simulink library "visionanalysis"  (R2024b)
settings: Solver=ode45  StartTime=0.0  StopTime=10.0  RelTol=1e-3
undefined symbols (not defined in the file or in its folder): dtInfo, fspecial
libraries: visionstatistics x1
(part 1 of 2)
settings Model: Creator=The MathWorks, Inc.  LastModifiedBy=The MathWorks, Inc.
settings SolverCC: AlgebraicLoopSolver=TrustRegion  MaxZcPerStep=1
settings DataIOCC: LimitDataPoints=on  SaveFormat=Array  SignalLoggingSaveFormat=ModelDataLogs  ReturnWorkspaceOutputs=off
settings OptimizationCC: BlockReduction=off  BooleanDataType=off  ReuseModelBlockBuffer=off  ExpressionDepthLimit=2147483647  EfficientMapNaN2IntZero=off  LifeSpan=inf
settings DebuggingCC: SaveWithParameterizedLinksMsg=none  UnderspecifiedInitializationDetection=Classic  MergeDetectMultiDrivingBlocksExec=none  SignalResolutionControl=TryResolveAllWithWarning  FcnCallInpInsideContextMsg=warning  UnconnectedInputMsg=warning  UnconnectedOutputMsg=warning  UnconnectedLineMsg=warning  AllowSymbolicDim=off  StateNameClashWarn=warning  SFUnexpectedBacktrackingDiag=warning  SFNoUnconditionalDefaultTransitionDiag=warning  SFExecutionAtInitializationDiag=none  ArithmeticOperatorsInVariantConditions=warning
settings HardwareCC: ProdBitPerPointer=32  ProdBitPerSizeT=32  ProdBitPerPtrDiffT=32  ProdLargestAtomicFloat=None  ProdIntDivRoundTo=Undefined  ProdEndianess=Unspecified  ProdWordSize=32  ProdHWDeviceType=32-bit Generic  TargetUnknown=on
settings ModelReferenceCC: EnableRefExpFcnMdlSchedulingChecks=on  PropagateSignalLabelsOutOfModel=off
settings SFSimCC: SimUseLocalCustomCode=off
settings RTWCC: RTWUseLocalCustomCode=off  GPUComputeCapability=3.5  DLArmComputeVersion=19.05
settings CodeAppCC: StateflowObjectComments=on
settings GRTTargetCC: TargetLangStandard=C89/C90 (ANSI)  CombineOutputUpdateFcns=off  GRTInterface=on
settings ConfigComp: CovMetricSettings=dw  CovSaveCumulativeToWorkspaceVar=on  CovSaveSingleToWorkspaceVar=on  CovExternalEMLEnable=off  CovSFcnEnable=off

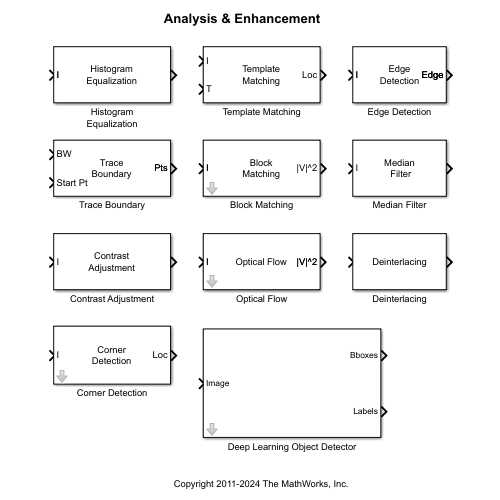
[thumbnail: Simulink's stored preview of the top-level diagram]
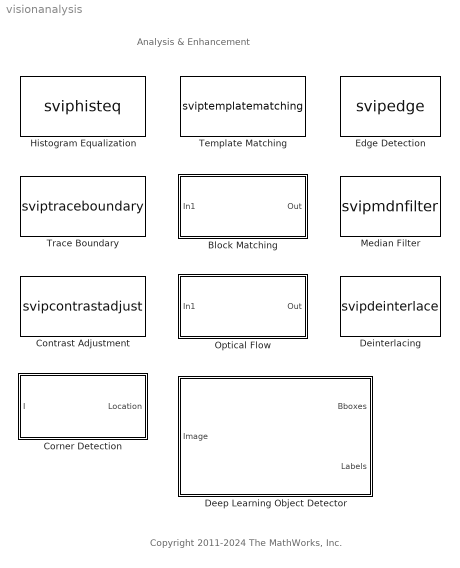
== system visionanalysis ==
  note: Analysis & Enhancement
  note: Copyright 2011-2024 The MathWorks, Inc.
  Block Matching : Subsystem  mask(Block Matching){which2img=Current frame and N-th frame back, N=1, searchMethod=Exhaustive, matchCriteria=Mean square error (MSE), blockSize=[17 17], overlapping=[0 0], maxDisplacement=[7 7], outVelForm=Magnitude-squared, roundingMode=Floor, overflowMode=on, prodOutputMode=Binary point scaling, prodOutputWordLength=32, prodOutputFracLength=0, accumMode=Binary point scaling, accumWordLength=32, accumFracLength=0, outputMode=Binary point scaling, outputWordLength=8, outputFracLength=0, LockScale=off}
      mask prompts: which2img "vision:masks:EstimateMotionBetween"; N "vision:masks:N"; searchMethod "vision:masks:SearchMethod"; matchCriteria "vision:masks:BlockMatchingCriteria"; blockSize "vision:masks:BlockSizeheightWidth"; overlapping "vision:masks:OverlapSizerC"; maxDisplacement "vision:masks:MaximumDisplacementrC"; outVelForm "vision:masks:VelocityOutput"; roundingMode "vision:masks:RoundingMode"; overflowMode "vision:masks:SaturateOnIntegerOverflow"; LockScale "Simulink:masks:LockDataTypeAgainstFxpTools_MP"
      mask help: vision:masks:BlockMatchingDescription
      mask init:
      | [disp_str,si,so]=vipblkblockmatch('icon',which2img);
      | vipblkblockmatch('init');
      mask Help: eval('visionblockhelp');
      mask TypeOptions which2img: vision:masks:TwoImages | vision:masks:CurrentFrameAndNthFrameBack
      mask Callback which2img: vipblkblockmatch('dynamic');
      mask TypeOptions searchMethod: vision:masks:Exhaustive | vision:masks:Threestep
      mask TypeOptions matchCriteria: vision:masks:MeanSquareErrorMSE | vision:masks:MeanAbsoluteDifferenceMAD
      mask Callback matchCriteria: vipblkblockmatch('dynamic');
      mask TypeOptions outVelForm: vision:masks:HorizontalAndVerticalComponentsI | vision:masks:Magnitudesquared
      mask Callback outVelForm: vipblkblockmatch('dynamic');
      mask TypeOptions roundingMode: Simulink:dialog:Ceiling_CB | Simulink:dialog:Convergent_CB | Simulink:dialog:Floor_CB | Simulink:dialog:Nearest_CB | Simulink:dialog:Round_CB | Simulink:dialog:Simplest_CB | Simulink:dialog:Zero_CB
      mask TypeOptions prodOutputMode: Simulink:dialog:UDTSameAsInputRule | vision:masks:BinaryPointScaling
      mask Callback prodOutputMode: vipblkblockmatch('dynamic');
      mask TypeOptions accumMode: vision:masks:BinaryPointScaling
      mask Callback accumMode: vipblkblockmatch('dynamic');
      mask TypeOptions outputMode: vision:masks:BinaryPointScaling
      mask Callback outputMode: vipblkblockmatch('dynamic');
      mask DialogControl MainTab Prompt: vision:masks:Main
      mask DialogControl which2img Prompt: Estimate motion between:
      mask DialogControl N Prompt: N:
      mask DialogControl searchMethod Prompt: Search method:
      mask DialogControl matchCriteria Prompt: Block matching criteria:
      mask DialogControl blockSize Prompt: Block size [height width]:
      mask DialogControl overlapping Prompt: Overlap size [r c]:
      mask DialogControl maxDisplacement Prompt: Maximum displacement [r c]:
      mask DialogControl outVelForm Prompt: Velocity output:
      mask DialogControl DataTypesTab Prompt: Simulink:dialog:DataTypesTab
      mask DialogControl FloatingPointTrumpRule Prompt: Simulink:dialog:FloatingPointTrumpRule
      mask DialogControl FixPtOpParamsGroupBox Prompt: vision:masks:FixptOpParams
      mask DialogControl roundingMode Prompt: Rounding mode:
      mask DialogControl overflowMode Prompt: Saturate on integer overflow
      mask DialogControl FixptDatatypesGroupBox Prompt: vision:masks:FixptDataTypes
      mask DialogControl DataTypeColumnLabel Prompt: Simulink:dialog:FcnColumnHeaderDataType
      mask DialogControl SignedColumnLabel Prompt: Simulink:dialog:UDTSignedSign
      mask DialogControl WordLengthColumnLabel Prompt: Simulink:dialog:UDTWordLengthEdit
      mask DialogControl FractionLengthColumnLabel Prompt: Simulink:dialog:UDTFractionLengthEdit
      mask DialogControl prodOutputLabel Prompt: Simulink:dialog:ProdPrompt
      mask DialogControl prodOutputSignedText Prompt: Simulink:dialog:yes_CB
      mask DialogControl accumLabel Prompt: Simulink:dialog:AccumPrompt
      mask DialogControl accumSignedText Prompt: dspshared:FixptDialog:yes
      mask DialogControl outputLabel Prompt: Simulink:dialog:OutputPrompt
      mask DialogControl outputSignedText Prompt: Simulink:dialog:no_CB
      mask DialogControl LockScale Prompt: Lock data type settings against changes by the fixed-point tools
      mask Display:
      | disp(disp_str);
      | port_label('input',si(1).port,si(1).txt);
      | port_label('input',si(2).port,si(2).txt);
      | 
      | port_label('output',1,so(1).txt);
  Contrast Adjustment : S-Function  FunctionName=svipcontrastadjust  Parameters=methodInputRange, rangeIn, fracSaturate, isBinNum, binNum, methodOutputRange, rangeOut, prod1Mode, prod1WordLength, prod1FracLength, prod2Mode, prod2WordLength, prod2FracLength, dtInfo.roundingMode, dtInfo.overflowMode  SFunctionDeploymentMode=off  EnableBusSupport=off  mask(Contrast Adjustment){methodInputRange=Full input data range [min max], rangeIn=[0 255], fracSaturate=[1 1], isBinNum=on, binNum=256, methodOutputRange=Full data type range, rangeOut=[0 255], roundingMode=Floor, overflowMode=off, prod1Mode=Binary point scaling, prod1WordLength=32, prod1FracLength=16, prod2Mode=Binary point scaling, prod2WordLength=32, prod2FracLength=16, LockScale=off}
      mask prompts: methodInputRange "vision:masks:AdjustPixelValuesFrom"; rangeIn "vision:masks:RangelowHigh"; fracSaturate "vision:masks:PercentageOfPixelsToSaturatelowH"; isBinNum "vision:masks:SpecifyNumberOfHistogramBinsused"; binNum "vision:masks:NumberOfHistogramBins"; methodOutputRange "vision:masks:AdjustPixelValuesTo"; rangeOut "vision:masks:RangelowHigh"; roundingMode "vision:masks:RoundingMode"; overflowMode "vision:masks:SaturateOnIntegerOverflow"; LockScale "Simulink:masks:LockDataTypeAgainstFxpTools_MP"
      mask help: vision:masks:ContrastAdjustmentDescription
      mask init:
      | dtInfo = dspGetFixptDataTypeInfo(gcbh,1);
      | fracSaturate = single(fracSaturate) ./ single(100);
      mask Help: eval('visionblockhelp');
      mask TypeOptions methodInputRange: vision:masks:FullInputDataRangeminMax | vision:masks:UserdefinedRange | vision:masks:RangeDeterminedBySaturating
      mask Callback methodInputRange: vipblkcontrast;
      mask Callback isBinNum: vipblkcontrast;
      mask TypeOptions methodOutputRange: vision:masks:FullDataTypeRange | vision:masks:UserdefinedRange
      mask Callback methodOutputRange: vipblkcontrast;
      mask TypeOptions roundingMode: Simulink:dialog:Ceiling_CB | Simulink:dialog:Convergent_CB | Simulink:dialog:Floor_CB | Simulink:dialog:Nearest_CB | Simulink:dialog:Round_CB | Simulink:dialog:Simplest_CB | Simulink:dialog:Zero_CB
      mask TypeOptions prod1Mode: vision:masks:BinaryPointScaling
      mask Callback prod1Mode: vipblkcontrast;
      mask TypeOptions prod2Mode: vision:masks:BinaryPointScaling
      mask Callback prod2Mode: vipblkcontrast;
      mask DialogControl mainTab Prompt: vision:masks:Main
      mask DialogControl methodInputRange Prompt: Adjust pixel values from:
      mask DialogControl rangeIn Prompt: Range [low high]:
      mask DialogControl fracSaturate Prompt: Percentage of pixels to saturate [low high]:
      mask DialogControl isBinNum Prompt: Specify number of histogram bins (used to calculate the range when outliers are eliminated)
      mask DialogControl binNum Prompt: Number of histogram bins:
      mask DialogControl methodOutputRange Prompt: Adjust pixel values to:
      mask DialogControl rangeOut Prompt: Range [low high]:
      mask DialogControl dataTypesTab Prompt: vision:masks:DataTypes
      mask DialogControl dataTypesDescription Prompt: Simulink:dialog:FloatingPointTrumpRule
      mask DialogControl fixedptOpParams Prompt: vision:masks:FixptOpParams
      mask DialogControl roundingMode Prompt: Rounding mode:
      mask DialogControl overflowMode Prompt: Saturate on integer overflow
      mask DialogControl fixedptDataTypes Prompt: vision:masks:FixptDataTypes
      mask DialogControl openDataTypeDiagram Prompt: vision:masks:OpenDataTypeDiagram
      mask DialogControl openDataTypeDiagram Callback: uiservices.helpview('$DOCROOT$\toolbox\vision\vision.map', 'contrastadjust', 'CSHelpWindow')
      mask DialogControl dataTypeColoumnLabel Prompt: Simulink:dialog:FcnColumnHeaderDataType
      mask DialogControl signedColoumnLabel Prompt: Simulink:dialog:UDTSignedSign
      mask DialogControl wordLegthColoumnlabel Prompt: Simulink:dialog:UDTWordLengthEdit
      mask DialogControl fracLengthColumnLabel Prompt: Simulink:dialog:UDTFractionLengthEdit
      mask DialogControl product1Label Prompt: vision:masks:Product1
      mask DialogControl prod1SignedText Prompt: Simulink:dialog:yes_CB
      mask DialogControl product2Label Prompt: vision:masks:Product2
      mask DialogControl prod2SignedText Prompt: Simulink:dialog:yes_CB
      mask DialogControl LockScale Prompt: Lock data type settings against changes by the fixed-point tools
      mask Display:
      | disp('Contrast\nAdjustment');
      | port_label('input',1,'I');
  Corner Detection : Subsystem  mask(Corner Detection){method=Harris corner detection (Harris & Stephens), factor=0.04, filter=fspecial('gaussian', [1 5], 1.5), thrInten=0.1, thrAngle=157.5, output=Obsolete9b, outputInUse=Corner location, maxNum=200, thrMetric=0.0005, neighborSize=[11 11], isOutVarDim=on, roundingMode=Floor, overflowMode=off, firstCoeffMode=Specify word length, firstCoeffWordLength=16, firstCoeffFracLength=16, prodOutputMode=Binary point scaling, prodOutputWordLength=32, prodOutputFracLength=0, accumMode=Binary point scaling, accumWordLength=32, accumFracLength=0, memoryMode=Binary point scaling, memoryWordLength=32, memoryFracLength=0, outputMode=Same as accumulator, outputWordLength=32, outputFracLength=0, LockScale=off}
      mask prompts: method "vision:masks:Method"; factor "vision:masks:SensitivityFactor"; filter "vision:masks:CoefficientsSeparableSmoothing"; thrInten "vision:masks:IntensityComparisonThreshold"; thrAngle "vision:masks:MaximumAngleToBeConsidered"; output "dspshared:FixptDialog:Output_MP"; outputInUse "dspshared:FixptDialog:Output_MP"; maxNum "vision:masks:MaximumNumberOfCorners"; thrMetric "vision:masks:MinimumMetricValueThatIndicates"; neighborSize "vision:masks:NeighborhoodSizesuppressRegion"; isOutVarDim "vision:masks:OutputVariableSizeSignal"; roundingMode "vision:masks:RoundingMode"; overflowMode "vision:masks:SaturateOnIntegerOverflow"; LockScale "Simulink:masks:LockDataTypeAgainstFxpTools_MP"
      mask help: vision:masks:CornerDetectionDescription
      mask init:
      | blkh = gcbh;
      | dtInfo = dspGetFixptDataTypeInfo(blkh, 63); %63
      | outport = vipblkcornerdetection(blkh, output, outputInUse, isOutVarDim);
      mask Help: eval('visionblockhelp');
      mask TypeOptions method: vision:masks:HarrisCornerDetectionHarrisSteph | vision:masks:MinimumEigenvalueShiTomasi | vision:masks:LocalIntensityComparisonRosenDr
      mask Callback method: vipblkcddynamic;
      mask TypeOptions thrAngle: 22.5 | 45.0 | 67.5 | 90.0 | 112.5 | 135.0 | 157.5
      mask TypeOptions output: vision:masks:CornerLocation | vision:masks:CornerLocationAndMetricMatrix | vision:masks:MetricMatrix | vision:masks:Obsolete9b
      mask TypeOptions outputInUse: vision:masks:CornerLocation | vision:masks:CornerLocationAndMetricMatrix | vision:masks:MetricMatrix
      mask Callback outputInUse: vipblkcddynamic;
      mask TypeOptions roundingMode: Simulink:dialog:Ceiling_CB | Simulink:dialog:Convergent_CB | Simulink:dialog:Floor_CB | Simulink:dialog:Nearest_CB | Simulink:dialog:Round_CB | Simulink:dialog:Simplest_CB | Simulink:dialog:Zero_CB
      mask TypeOptions firstCoeffMode: Simulink:dialog:UDTSameAsInputWordLengthRule | vision:masks:SpecifyWordLength | vision:masks:BinaryPointScaling
      mask Callback firstCoeffMode: vipblkcddynamic;
      mask TypeOptions prodOutputMode: Simulink:dialog:UDTSameAsInputRule | vision:masks:BinaryPointScaling
      mask Callback prodOutputMode: vipblkcddynamic;
      mask TypeOptions accumMode: Simulink:dialog:UDTSameAsInputRule | vision:masks:BinaryPointScaling
      mask Callback accumMode: vipblkcddynamic;
      mask TypeOptions memoryMode: Simulink:dialog:UDTSameAsInputRule | vision:masks:BinaryPointScaling
      mask Callback memoryMode: vipblkcddynamic;
      mask TypeOptions outputMode: Simulink:dialog:UDTSameAsAccumulatorRule | Simulink:dialog:UDTSameAsInputRule | vision:masks:BinaryPointScaling
      mask Callback outputMode: vipblkcddynamic;
      mask DialogControl maintab Prompt: vision:masks:Main
      mask DialogControl method Prompt: Method:
      mask DialogControl factor Prompt: Sensitivity factor (0<k<0.25):
      mask DialogControl filter Prompt: Coefficients for separable smoothing filter:
      mask DialogControl thrInten Prompt: Intensity comparison threshold:
      mask DialogControl thrAngle Prompt: Maximum angle to be considered a corner (in degrees):
      mask DialogControl output Prompt: Output:
      mask DialogControl outputInUse Prompt: Output:
      mask DialogControl maxNum Prompt: Maximum number of corners:
      mask DialogControl thrMetric Prompt: Minimum metric value that indicates a corner:
      mask DialogControl neighborSize Prompt: Neighborhood size (suppress region around detected corners):
      mask DialogControl isOutVarDim Prompt: Output variable size signal
      mask DialogControl dataTypesTab Prompt: vision:masks:DataTypes
      mask DialogControl fixptTrumpRule Prompt: Simulink:dialog:FloatingPointTrumpRule
      mask DialogControl fixptOpParams Prompt: vision:masks:FixptOpParams
      mask DialogControl roundingMode Prompt: Rounding mode:
      mask DialogControl overflowMode Prompt: Saturate on integer overflow
      mask DialogControl fixptDataTypes Prompt: vision:masks:FixptDataTypes
      mask DialogControl openDataTypeDiagram Prompt: vision:masks:OpenDataTypeDiagram
      mask DialogControl openDataTypeDiagram Callback: uiservices.helpview('$DOCROOT$\toolbox\vision\vision.map', 'cornerdetection', 'CSHelpWindow')
      mask DialogControl dataTypeColumnLabel Prompt: Simulink:dialog:FcnColumnHeaderDataType
      mask DialogControl signedColumnLabel Prompt: Simulink:dialog:UDTSignedSign
      mask DialogControl wordLengthColumnLabel Prompt: Simulink:dialog:UDTWordLengthEdit
      mask DialogControl fractionLengthColumnLabel Prompt: Simulink:dialog:UDTFractionLengthEdit
      mask DialogControl firstCoeffLabel Prompt: vision:masks:Coefficients
      mask DialogControl firstCoeffSignedText Prompt: Simulink:dialog:Yes_CB
      mask DialogControl prodOutputLabel Prompt: vision:masks:ProductOutput
      mask DialogControl prodOutputSignedText Prompt: Simulink:dialog:Yes_CB
      mask DialogControl accumLabel Prompt: vision:masks:Accumulator
      mask DialogControl accumSignedText Prompt: Simulink:dialog:Yes_CB
      mask DialogControl memoryLabel Prompt: vision:masks:Memory
      mask DialogControl memorySignedText Prompt: Simulink:dialog:Yes_CB
      mask DialogControl outputLabel Prompt: vision:masks:MetricOutput
      mask DialogControl outputSignedText Prompt: Simulink:dialog:Yes_CB
      mask DialogControl LockScale Prompt: Lock data type settings against changes by the fixed-point tools
      mask Display:
      | disp('Corner\nDetection');
      | port_label('input',1,'I');
      | port_label('output', outport(1).port, outport(1).txt);
      | port_label('output', outport(2).port, outport(2).txt);
      | port_label('output', outport(3).port, outport(3).txt);
  Deep Learning Object Detector : Subsystem  mask(Deep Learning Object Detector){Detector=Detector from MAT-file, DetectorFunction=untitled, DetectorFilePath=untitled.mat, MaxDetections=500, Bboxes=on, Labels=on, Scores=off, UseROI=off, AutoResize=on, ROI=[1 1 100 100], Threshold=0.5, NumStrongestRegions=2000, UseMinSize=off, MinSize=[1 1], UseMaxSize=off, MaxSize=[50 50], ForceInterpretedSim=off}
      mask prompts: Detector "vision:ObjectDetectorBlock:Detector"; DetectorFunction "vision:ObjectDetectorBlock:MatlabFunction"; DetectorFilePath "vision:ObjectDetectorBlock:FilePath"; MaxDetections "vision:ObjectDetectorBlock:MaxDetections"; Bboxes "vision:ObjectDetectorBlock:Bboxes"; Labels "vision:ObjectDetectorBlock:Labels"; Scores "vision:ObjectDetectorBlock:Scores"; UseROI "vision:ObjectDetectorBlock:UseROI"; AutoResize "Automatically resize input"; Threshold "vision:ObjectDetectorBlock:Threshold"; NumStrongestRegions "vision:ObjectDetectorBlock:NumStrongestRegions"; UseMinSize "vision:ObjectDetectorBlock:UseMinSize"; UseMaxSize "vision:ObjectDetectorBlock:UseMaxSize"; ForceInterpretedSim "vision:ObjectDetectorBlock:ForceInterpretedSim"
      mask help: vision:ObjectDetectorBlock:Description
      mask init:
      | vision.internal.blocks.objectDetectorBlockWrapper(...
      |     'deep.blocks.internal.configureObjectDetector', ...
      |     gcb, ...
      |     bdroot, ...
      |     Detector, ...
      |     DetectorFilePath, ...
      |     DetectorFunction, ...
      |     logical(UseROI), ...
      |     ROI, ...
      |     Threshold, ...
      |     NumStrongestRegions, ...
      |     logical(AutoResize), ...
      |     logical(UseMinSize), ...
      |     MinSize, ...
      |     logical(UseMaxSize), ...
      |     MaxSize, ...
      |     MaxDetections, ...
      |     logical(Bboxes), ...
      |     logical(Labels), ...
      |     logical(Scores), ...
      |     logical(ForceInterpretedSim));
      mask Help: helpview('vision', 'nnet_model_detect')
      mask TypeOptions Detector: vision:ObjectDetectorBlock:DetectorFromMatFile | vision:ObjectDetectorBlock:DetectorFromFunction
      mask Callback Detector: vision.internal.blocks.objectDetectorBlockWrapper('deep.blocks.internal.setNetworkSelectVisibility',gcb);
      mask Callback DetectorFunction: vision.internal.blocks.objectDetectorBlockWrapper('deep.blocks.internal.setObjectDetectorOptionsVisibility', gcb);
      mask Callback DetectorFilePath: vision.internal.blocks.objectDetectorBlockWrapper('deep.blocks.internal.setObjectDetectorOptionsVisibility', gcb);
      mask Callback UseROI: vision.internal.blocks.objectDetectorBlockWrapper('deep.blocks.internal.setEnabledParameterVisibility', gcb, 'UseROI', 'ROI');
      mask Callback UseMinSize: vision.internal.blocks.objectDetectorBlockWrapper('deep.blocks.internal.setEnabledParameterVisibility', gcb, 'UseMinSize', 'MinSize');
      mask Callback UseMaxSize: vision.internal.blocks.objectDetectorBlockWrapper('deep.blocks.internal.setEnabledParameterVisibility', gcb, 'UseMaxSize', 'MaxSize');
      mask DialogControl Detector Prompt: Detector:
      mask DialogControl DetectorFunction Prompt: MATLAB function:
      mask DialogControl DetectorFilePath Prompt: File path:
      mask DialogControl BrowseButton Prompt: vision:ObjectDetectorBlock:Browse
      mask DialogControl BrowseButton Callback: vision.internal.blocks.objectDetectorBlockWrapper('deep.blocks.internal.handleBrowseButtonClick', gcb);
      mask DialogControl OutputsTab Prompt: vision:ObjectDetectorBlock:Outputs
      mask DialogControl OutputsSizeGroup Prompt: vision:ObjectDetectorBlock:OutputsSize
      mask DialogControl MaxDetections Prompt: Maximum number of detections:
      mask DialogControl OutputPortsGroup Prompt: vision:ObjectDetectorBlock:OutputPorts
      mask DialogControl Bboxes Prompt: Bounding boxes
      mask DialogControl AdvancedTab Prompt: vision:ObjectDetectorBlock:Advanced
      mask DialogControl AdvancedParametersGroup Prompt: vision:ObjectDetectorBlock:AdvancedParameters
      mask DialogControl UseROI Prompt: Specify region of interest
      mask DialogControl Threshold Prompt: Detection threshold:
      mask DialogControl NumStrongestRegions Prompt: Number of strongest regions:
      mask DialogControl UseMinSize Prompt: Specify minimum region size
      mask DialogControl UseMaxSize Prompt: Specify maximum region size
      mask DialogControl HiddenContainer Prompt: Hidden Parameters
      mask DialogControl ForceInterpretedSim Prompt: Force interpreted simulation
  Deinterlacing : S-Function  FunctionName=svipdeinterlace  Parameters=method,isInputTransposed,dtInfo.accumMode,dtInfo.accumWordLength,dtInfo.accumFracLength,dtInfo.outputMode,dtInfo.outputWordLength,dtInfo.outputFracLength,dtInfo.roundingMode,dtInfo.overflowMode  SFunctionDeploymentMode=off  EnableBusSupport=off  mask(Deinterlacing){method=Line repetition, isInputTransposed=off, roundingMode=Floor, overflowMode=on, prodOutputMode=Same as input, prodOutputWordLength=12, prodOutputFracLength=3, accumMode=Binary point scaling, accumWordLength=12, accumFracLength=3, outputMode=Same as input, outputWordLength=8, outputFracLength=0, LockScale=off}
      mask prompts: method "vision:masks:Method"; isInputTransposed "vision:masks:InputImageIsTransposed"; roundingMode "vision:masks:RoundingMode"; overflowMode "vision:masks:SaturateOnIntegerOverflow"; LockScale "Simulink:masks:LockDataTypeAgainstFxpTools_MP"
      mask help: vision:masks:DeinterlacingDescription
      mask init:
      | dtInfo = dspGetFixptDataTypeInfo(gcbh,7);
      | vipblkdeinterlacing('dynamic');
      mask Help: eval('visionblockhelp');
      mask TypeOptions method: vision:masks:LineRepetition | vision:masks:LinearInterpolation | vision:masks:VerticalTemporalMedianFiltering
      mask Callback method: vipblkdeinterlacing('dynamic');
      mask TypeOptions roundingMode: Simulink:dialog:Ceiling_CB | Simulink:dialog:Convergent_CB | Simulink:dialog:Floor_CB | Simulink:dialog:Nearest_CB | Simulink:dialog:Round_CB | Simulink:dialog:Simplest_CB | Simulink:dialog:Zero_CB
      mask TypeOptions prodOutputMode: Simulink:dialog:UDTSameAsInputRule | vision:masks:BinaryPointScaling
      mask Callback prodOutputMode: vipblkdeinterlacing('dynamic');
      mask TypeOptions accumMode: Simulink:dialog:UDTSameAsInputRule | vision:masks:BinaryPointScaling
      mask Callback accumMode: vipblkdeinterlacing('dynamic');
      mask TypeOptions outputMode: Simulink:dialog:UDTSameAsInputRule | vision:masks:BinaryPointScaling
      mask Callback outputMode: vipblkdeinterlacing('dynamic');
      mask DialogControl MainTab Prompt: vision:masks:Main
      mask DialogControl method Prompt: Method:
      mask DialogControl isInputTransposed Prompt: Input image is transposed (data order is row major)
      mask DialogControl DataTypesTab Prompt: Simulink:dialog:DataTypesTab
      mask DialogControl emptyFixpt Prompt: vision:masks:FixedpointParametersLinearInterp
      mask DialogControl FloatingPointTrumpRule Prompt: Simulink:dialog:FloatingPointTrumpRule
      mask DialogControl FixPtOpParamsGroupBox Prompt: dspshared:FixptDialog:fixptOpParams
      mask DialogControl roundingMode Prompt: Rounding mode:
      mask DialogControl overflowMode Prompt: Saturate on integer overflow
      mask DialogControl FixptDatatypesGroupBox Prompt: dspshared:FixptDialog:fixptDataTypes
      mask DialogControl DataTypeColumnLabel Prompt: Simulink:dialog:BreakPointTableHeaderDT
      mask DialogControl SignedColumnLabel Prompt: dspshared:FixptDialog:signed
      mask DialogControl WordLengthColumnLabel Prompt: dspshared:FixptDialog:wordLength
      mask DialogControl FractionLengthColumnLabel Prompt: dspshared:FixptDialog:fractionLength
      mask DialogControl prodOutputLabel Prompt: Simulink:dialog:ProdPrompt
      mask DialogControl prodOutputSignedText Prompt: Simulink:dialog:UDTSameAsInputRule
      mask DialogControl accumLabel Prompt: Simulink:dialog:AccumPrompt
      mask DialogControl accumSignedText Prompt: Simulink:dialog:UDTSameAsInputRule
      mask DialogControl outputLabel Prompt: Simulink:dialog:OutputPrompt
      mask DialogControl outputSignedText Prompt: Simulink:dialog:UDTSameAsInputRule
      mask DialogControl LockScale Prompt: Lock data type settings against changes by the fixed-point tools
      mask Display: disp('Deinterlacing')
  Edge Detection : S-Function  FunctionName=svipedge  Parameters=method, outputType, userDefinedThreshold, thresholdSource, threshold, thresholdTuning, edgeThinning,threshold_canny,autoPercent,sigma,dtInfo. prodOutputMode,dtInfo.prodOutputWordLength,dtInfo.prodOutputFracLength,dtInfo.accumMode,dtInfo.accumWordLength,dtInfo.accumFracLength,dtInfo.outputMode,dtInfo.outputWordLength,dtInfo.outputFracLength,dtInfo.roundingMode,dtInfo.overflowMode  SFunctionDeploymentMode=off  EnableBusSupport=off  mask(Edge Detection){method=Sobel, outputType=Binary image, userDefinedThreshold=off, thresholdSource=Input port, threshold=20, thresholdTuning=4, edgeThinning=off, threshold_canny=[0.25 0.60], autoPercent=70, sigma=1, roundingMode=Floor, overflowMode=off, prodOutputMode=Binary point scaling, prodOutputWordLength=32, prodOutputFracLength=8, accumMode=Same as first input, accumWordLength=32, accumFracLength=8, outputMode=Same as first input, outputWordLength=16, outputFracLength=4, LockScale=off}
      mask prompts: method "vision:masks:Method"; outputType "vision:masks:OutputType"; userDefinedThreshold "vision:masks:UserdefinedThreshold"; thresholdSource "vision:masks:ThresholdSource"; threshold "vision:masks:Threshold"; thresholdTuning "vision:masks:ThresholdScaleFactor"; edgeThinning "vision:masks:EdgeThinning"; threshold_canny "vision:masks:ThresholdLowHigh"; autoPercent "vision:masks:ApproximatePercentageOfWeakEdge"; sigma "vision:masks:StandardDeviationOfGaussian"; roundingMode "vision:masks:RoundingMode"; overflowMode "vision:masks:SaturateOnIntegerOverflow"; LockScale "Simulink:masks:LockDataTypeAgainstFxpTools_MP"
      mask help: vision:masks:EdgeDetectionDescription
      mask init:
      | [si,so,blkname,dtInfo]= vipblkedge('init');
      mask Help: eval('visionblockhelp');
      mask TypeOptions method: vision:masks:Sobel | vision:masks:Prewitt | vision:masks:Roberts | vision:masks:Canny
      mask Callback method: vipblkedge('dynamic');
      mask TypeOptions outputType: vision:masks:BinaryImage | vision:masks:GradientComponents | vision:masks:BinaryImageAndGradientComponents
      mask Callback outputType: vipblkedge('dynamic');
      mask Callback userDefinedThreshold: vipblkedge('dynamic');
      mask TypeOptions thresholdSource: vision:masks:SpecifyViaDialog | vision:masks:InputPort
      mask Callback thresholdSource: vipblkedge('dynamic');
      mask TypeOptions roundingMode: Simulink:dialog:Ceiling_CB | Simulink:dialog:Convergent_CB | Simulink:dialog:Floor_CB | Simulink:dialog:Nearest_CB | Simulink:dialog:Round_CB | Simulink:dialog:Simplest_CB | Simulink:dialog:Zero_CB
      mask TypeOptions prodOutputMode: Simulink:dialog:UDTSameAsFirstInputRule | vision:masks:BinaryPointScaling
      mask Callback prodOutputMode: vipblkedge('dynamic');
      mask TypeOptions accumMode: Simulink:dialog:UDTSameAsProductRule | Simulink:dialog:UDTSameAsFirstInputRule | vision:masks:BinaryPointScaling
      mask Callback accumMode: vipblkedge('dynamic');
      mask TypeOptions outputMode: Simulink:dialog:UDTSameAsAccumulatorRule | Simulink:dialog:UDTSameAsProductRule | Simulink:dialog:UDTSameAsFirstInputRule | vision:masks:BinaryPointScaling
      mask Callback outputMode: vipblkedge('dynamic');
      mask DialogControl MainTab Prompt: vision:masks:Main
      mask DialogControl method Prompt: Method:
      mask DialogControl outputType Prompt: Output type:
      mask DialogControl userDefinedThreshold Prompt: User-defined threshold
      mask DialogControl thresholdSource Prompt: Threshold source:
      mask DialogControl threshold Prompt: Threshold:
      mask DialogControl thresholdTuning Prompt: Threshold scale factor:(used to automatically calculate threshold value)
      mask DialogControl edgeThinning Prompt: Edge thinning
      mask DialogControl threshold_canny Prompt: Threshold, [Low High]:
      mask DialogControl autoPercent Prompt: Approximate percentage of weak edge and nonedge pixels:(used to automatically calculate threshold values)
      mask DialogControl sigma Prompt: Standard deviation of Gaussian filter:
      mask DialogControl DataTypesTab Prompt: Simulink:dialog:DataTypesTab
      mask DialogControl emptyFixpt Prompt: vision:masks:FixedpointInputIsNotSupported
      mask DialogControl FloatingPointTrumpRule Prompt: Simulink:dialog:FloatingPointTrumpRule
      mask DialogControl FixPtOpParamsGroupBox Prompt: dspshared:FixptDialog:fixptOpParams
      mask DialogControl roundingMode Prompt: Rounding mode:
      mask DialogControl overflowMode Prompt: Saturate on integer overflow
      mask DialogControl FixptDatatypesGroupBox Prompt: dspshared:FixptDialog:fixptDataTypes
      mask DialogControl DataTypeColumnLabel Prompt: Simulink:dialog:BreakPointTableHeaderDT
      mask DialogControl SignedColumnLabel Prompt: dspshared:FixptDialog:signed
      mask DialogControl WordLengthColumnLabel Prompt: dspshared:FixptDialog:wordLength
      mask DialogControl FractionLengthColumnLabel Prompt: dspshared:FixptDialog:fractionLength
      mask DialogControl prodOutputLabel Prompt: Simulink:dialog:ProdPrompt
      mask DialogControl prodOutputSignedText Prompt: dspshared:FixptDialog:yes
      mask DialogControl accumLabel Prompt: Simulink:dialog:AccumPrompt
      mask DialogControl accumSignedText Prompt: dspshared:FixptDialog:yes
      mask DialogControl outputLabel Prompt: vision:masks:Gradients
      mask DialogControl outputSignedText Prompt: dspshared:FixptDialog:yes
      mask DialogControl LockScale Prompt: Lock data type settings against changes by the fixed-point tools
      mask Display:
      | disp(blkname)
      | 
      | port_label('input', si(1).port, si(1).txt);
      | port_label('input', si(2).port, si(2).txt);
      | 
      | port_label('output',so(1).port, so(1).txt);
      | port_label('output',so(2).port, so(2).txt);
      | port_label('output',so(3).port, so(3).txt);
  Histogram Equalization : S-Function  FunctionName=sviphisteq  Parameters=specify, numbins, src, hist  SFunctionDeploymentMode=off  EnableBusSupport=off  mask(Histogram Equalization){specify=Uniform, numbins=64, src=Specify via dialog, hist=ones(1,64)}
      mask prompts: specify "vision:masks:TargetHistogram"; numbins "vision:masks:NumberOfBins"; src "vision:masks:HistogramSource"; hist "vision:masks:Histogram"
      mask help: vision:masks:HistogramEqualizationDescription
      mask init:
      | ports(1).num = 1;
      | ports(1).txt = 'I';
      | if (specify == 2 && src == 2)
      | 	ports(2).num = 2;
      | 	ports(2).txt = 'Hist';
      | else
      | 	ports(2).num = 1;
      | 	ports(2).txt = 'I';
      | end
      mask Help: eval('visionblockhelp');
      mask TypeOptions specify: vision:masks:Uniform | vision:masks:Userdefined
      mask Callback specify:
      | if (strcmp(get_param(gcbh,'specify'),'Uniform'))
      | 	set_param(gcbh,'MaskVisibilities',{'on','on','off','off'});
      | else
      | 	if (strcmp(get_param(gcbh,'src'),'Input port'))
      | 		set_param(gcbh,'MaskVisibilities',{'on','off','on','off'});
      | 	else
      | 		set_param(gcbh,'MaskVisibilities',{'on','off','on','on'});
      | 	end
      | end
      mask TypeOptions src: vision:masks:SpecifyViaDialog | vision:masks:InputPort
      mask Callback src:
      | if (strcmp(get_param(gcbh,'specify'),'User-defined'))
      | 	if (strcmp(get_param(gcbh,'src'),'Input port'))
      | 		set_param(gcbh,'MaskVisibilities',{'on','off','on','off'});
      | 	else
      | 		set_param(gcbh,'MaskVisibilities',{'on','off','on','on'});
      | 	end
      | end
      mask Display:
      | disp('Histogram\nEqualization');
      | 
      | port_label('input',ports(1).num,ports(1).txt);
      | port_label('input',ports(2).num,ports(2).txt);
  Median Filter : S-Function  FunctionName=svipmdnfilter  Parameters=nghbood,outSize,padType,padSrc,padVal,dtInfo.accumMode,dtInfo.accumWordLength,dtInfo.accumFracLength,dtInfo.outputMode,dtInfo.outputWordLength,dtInfo.outputFracLength,dtInfo.roundingMode,dtInfo.overflowMode  SFunctionDeploymentMode=off  EnableBusSupport=on  mask(Median Filter){nghbood=[3 3], outSize=Same as input port I, padType=Constant, padSrc=Specify via dialog, padVal=0, roundingMode=Floor, overflowMode=off, prodOutputMode=Same as input, prodOutputWordLength=32, prodOutputFracLength=30, accumMode=Same as input, accumWordLength=32, accumFracLength=30, outputMode=Same as input, outputWordLength=16, outputFracLength=15, LockScale=off}
      mask prompts: nghbood "vision:masks:NeighborhoodSize"; outSize "vision:masks:OutputSize"; padType "vision:masks:PaddingOptions"; padSrc "vision:masks:PadValueSource"; padVal "vision:masks:PadValue"; roundingMode "vision:masks:RoundingMode"; overflowMode "vision:masks:SaturateOnIntegerOverflow"; LockScale "Simulink:masks:LockDataTypeAgainstFxpTools_MP"
      mask help: vision:masks:MedianFilterDescription
      mask init:
      | [ports,dtInfo] = vipblkmdnfilter;
      mask Help: eval('visionblockhelp');
      mask Callback nghbood: vipblkmdnfilter;
      mask TypeOptions outSize: vision:masks:SameAsInputPortI | vision:masks:Valid
      mask Callback outSize: vipblkmdnfilter;
      mask TypeOptions padType: vision:masks:Constant | vision:masks:Replicate | vision:masks:Symmetric | vision:masks:Circular
      mask Callback padType: vipblkmdnfilter;
      mask TypeOptions padSrc: vision:masks:SpecifyViaDialog | vision:masks:InputPort
      mask Callback padSrc: vipblkmdnfilter;
      mask Callback padVal: vipblkmdnfilter;
      mask TypeOptions roundingMode: Simulink:dialog:Ceiling_CB | Simulink:dialog:Convergent_CB | Simulink:dialog:Floor_CB | Simulink:dialog:Nearest_CB | Simulink:dialog:Round_CB | Simulink:dialog:Simplest_CB | Simulink:dialog:Zero_CB
      mask TypeOptions prodOutputMode: Simulink:dialog:UDTSameAsInputRule | vision:masks:BinaryPointScaling
      mask TypeOptions accumMode: Simulink:dialog:UDTSameAsInputRule | vision:masks:BinaryPointScaling
      mask Callback accumMode: vipblkmdnfilter;
      mask TypeOptions outputMode: Simulink:dialog:UDTSameAsInputRule | vision:masks:BinaryPointScaling
      mask Callback outputMode: vipblkmdnfilter;
      mask DialogControl mainTab Prompt: vision:masks:Main
      mask DialogControl nghbood Prompt: Neighborhood size:
      mask DialogControl outSize Prompt: Output size:
      mask DialogControl padType Prompt: Padding options:
      mask DialogControl padSrc Prompt: Pad value source:
      mask DialogControl padVal Prompt: Pad value:
      mask DialogControl dataTypesTab Prompt: vision:masks:DataTypes
      mask DialogControl floatingPointTrumpRule Prompt: Simulink:dialog:FloatingPointTrumpRule
      mask DialogControl fixptOperationalParamsGroupBox Prompt: vision:masks:FixptOpParams
      mask DialogControl roundingMode Prompt: Rounding mode:
      mask DialogControl overflowMode Prompt: Saturate on integer overflow
      mask DialogControl fixedPtDataTypesGroupBox Prompt: vision:masks:FixptDataTypes
      mask DialogControl dataTypeColoumnLabel Prompt: Simulink:dialog:FcnColumnHeaderDataType
      mask DialogControl signedColoumnLabel Prompt: Simulink:dialog:UDTSignedSign
      mask DialogControl wordLegthColoumnlabel Prompt: Simulink:dialog:UDTWordLengthEdit
      mask DialogControl fracLengthColumnLabel Prompt: Simulink:dialog:UDTFractionLengthEdit
      mask DialogControl prodOutputLabel Prompt: vision:masks:ProductOutput
      mask DialogControl prodOutputSignedText Prompt: Simulink:dialog:UDTSameAsInputSign
      mask DialogControl accumLabel Prompt: vision:masks:Accumulator
      mask DialogControl accumSignedText Prompt: Simulink:dialog:UDTSameAsInputSign
      mask DialogControl outputLabel Prompt: vision:masks:Output
      mask DialogControl outputSignedText Prompt: Simulink:dialog:UDTSameAsInputSign
      mask DialogControl LockScale Prompt: Lock data type settings against changes by the fixed-point tools
      mask DialogControl whenBothAreOdd Prompt: vision:masks:WhenBothNeighborhoodDimensions
      mask Display:
      | disp('Median\n Filter');
      | port_label('input',ports.port1, ports.txt1);
      | port_label('input',ports.port2, ports.txt2);
      | port_label('output',ports.port3, ports.txt3);
  Optical Flow : Subsystem  mask(Optical Flow){method=Horn-Schunck, gradMethod=Difference filter [-1 1], which2img=Current frame and N-th frame back, N=1, lambda=1, numInports=3, sigmaS=1.5, sigmaW=1, discardNormalFlow=off, outputCurrentImage=off, stop_criteria=When maximum number of iterations is reached, maxIter=10, maxAllowAbsDiff=eps, outVelForm=Magnitude-squared, eigTh=0.0039, roundingMode=Nearest, overflowMode=on, prodOutputMode=Binary point scaling, prodOutputWordLength=32, prodOutputFracLength=20, accumMode=Same as product output, accumWordLength=32, accumFracLength=20, memoryMode=Same as accumulator, memoryWordLength=32, memoryFracLength=20, firstCoeffMode=Same word length as first input, firstCoeffWordLength=16, firstCoeffFracLength=12, outputMode=Binary point scaling, outputWordLength=32, outputFracLength=20, LockScale=off}
      mask prompts: method "vision:masks:Method"; gradMethod "vision:masks:TemporalGradientFilter"; which2img "vision:masks:ComputeOpticalFlowBetween"; N "vision:masks:N"; lambda "vision:masks:SmoothnessFactor"; numInports "vision:masks:NumberOfInputFramesToBuffer"; sigmaS "vision:masks:SDForImageSmoothing"; sigmaW "vision:masks:SDForGradientSmoothing"; discardNormalFlow "vision:masks:DiscardNormalFlowEstimates"; outputCurrentImage "vision:masks:OutputImageCorrespondingToMotion"; stop_criteria "vision:masks:StopIterativeSolution"; maxIter "vision:masks:MaximumNumberOfIterations"; maxAllowAbsDiff "vision:masks:VelocityDifferenceThreshold"; outVelForm "vision:masks:VelocityOutput"; eigTh "vision:masks:ThresholdForNoiseReduction"; roundingMode "vision:masks:RoundingMode"; overflowMode "vision:masks:SaturateOnIntegerOverflow"; LockScale "Simulink:masks:LockDataTypeAgainstFxpTools_MP"
      mask help: vision:masks:OpticalFlowDescription
      mask init:
      | [disp_str,si,so]=vipblkopticalflow(which2img,double(numInports));
      mask Help: eval('visionblockhelp');
      mask TypeOptions method: vision:masks:HornSchunck | vision:masks:LucasKanade
      mask Callback method: vipblkopticalflowDynamic;
      mask TypeOptions gradMethod: vision:masks:DerivativeOfGaussian | vision:masks:DifferenceFilter
      mask Callback gradMethod: vipblkopticalflowDynamic;
      mask TypeOptions which2img: vision:masks:TwoImages | vision:masks:CurrentFrameAndNthFrameBack
      mask Callback which2img: vipblkopticalflowDynamic;
      mask TypeOptions stop_criteria: vision:masks:WhenVelocityDifferenceFallsBelow | vision:masks:WhenMaximumNumberOfIterations | vision:masks:WhicheverComesFirst
      mask Callback stop_criteria: vipblkopticalflowDynamic;
      mask TypeOptions outVelForm: vision:masks:HorizontalAndVerticalComponentsI | vision:masks:Magnitudesquared
      mask Callback outVelForm: vipblkopticalflowDynamic;
      mask TypeOptions roundingMode: Simulink:dialog:Ceiling_CB | Simulink:dialog:Convergent_CB | Simulink:dialog:Floor_CB | Simulink:dialog:Nearest_CB | Simulink:dialog:Round_CB | Simulink:dialog:Simplest_CB | Simulink:dialog:Zero_CB
      mask TypeOptions prodOutputMode: vision:masks:BinaryPointScaling
      mask Callback prodOutputMode: vipblkopticalflowDynamic;
      mask TypeOptions accumMode: Simulink:dialog:UDTSameAsProductRule | vision:masks:BinaryPointScaling
      mask Callback accumMode: vipblkopticalflowDynamic;
      mask TypeOptions memoryMode: Simulink:dialog:UDTSameAsAccumulatorRule | Simulink:dialog:UDTSameAsProductRule | vision:masks:BinaryPointScaling
      mask Callback memoryMode: vipblkopticalflowDynamic;
      mask TypeOptions firstCoeffMode: dspshared:FixptDialog:SameWordLengthAsFirstInput | vision:masks:SpecifyWordLength | vision:masks:BinaryPointScaling
      mask Callback firstCoeffMode: vipblkopticalflowDynamic;
      mask TypeOptions outputMode: vision:masks:BinaryPointScaling
      mask Callback outputMode: vipblkopticalflowDynamic;
      mask DialogControl mainTab Prompt: vision:masks:Main
      mask DialogControl method Prompt: Method:
      mask DialogControl gradMethod Prompt: Temporal gradient filter:
      mask DialogControl which2img Prompt: Compute optical flow between:
      mask DialogControl N Prompt: N:
      mask DialogControl lambda Prompt: Smoothness factor:
      mask DialogControl numInports Prompt: Number of input frames to buffer:
      mask DialogControl sigmaS Prompt: Standard deviation for image smoothing filter:
      mask DialogControl sigmaW Prompt: Standard deviation for gradient smoothing filter:
      mask DialogControl discardNormalFlow Prompt: Discard normal flow estimates when constraint equation is ill-conditioned
      mask DialogControl outputCurrentImage Prompt: Output image corresponding to motion vectors (accounts for block delay)
      mask DialogControl stop_criteria Prompt: Stop iterative solution:
      mask DialogControl maxIter Prompt: Maximum number of iterations:
      mask DialogControl maxAllowAbsDiff Prompt: Velocity difference threshold:
      mask DialogControl outVelForm Prompt: Velocity output:
      mask DialogControl eigTh Prompt: Threshold for noise reduction:
      mask DialogControl dataTypesTab Prompt: vision:masks:DataTypes
      mask DialogControl fixedptOpParams Prompt: vision:masks:FixptOpParams
      mask DialogControl roundingMode Prompt: Rounding mode:
      mask DialogControl overflowMode Prompt: Saturate on integer overflow
      mask DialogControl fixedptDataTypes Prompt: vision:masks:FixptDataTypes
      mask DialogControl dataTypeColoumnLabel Prompt: Simulink:dialog:FcnColumnHeaderDataType
      mask DialogControl signedColoumnLabel Prompt: Simulink:dialog:UDTSignedSign
      mask DialogControl wordLegthColoumnlabel Prompt: Simulink:dialog:UDTWordLengthEdit
      mask DialogControl fracLengthColumnLabel Prompt: Simulink:dialog:UDTFractionLengthEdit
      mask DialogControl prodOutputLabel Prompt: vision:masks:ProductOutput
      mask DialogControl prodOutputSignedText Prompt: Simulink:dialog:yes_CB
      mask DialogControl accumLabel Prompt: vision:masks:Accumulator
      mask DialogControl accumSignedText Prompt: Simulink:dialog:yes_CB
      mask DialogControl memoryLabel Prompt: vision:masks:Gradients
      mask DialogControl memorySignedText Prompt: Simulink:dialog:yes_CB
      mask DialogControl firstCoeffLabel Prompt: vision:masks:Threshold
      mask DialogControl firstCoeffSignedText Prompt: Simulink:dialog:yes_CB
      mask DialogControl outputLabel Prompt: vision:masks:Output
      mask DialogControl outputSignedText Prompt: Simulink:dialog:No_CB
      mask DialogControl LockScale Prompt: Lock data type settings against changes by the fixed-point tools
      mask DialogControl noDataTypes Prompt: vision:masks:FixedpointInputSupportedLucasKanade
      mask Display:
      | disp(disp_str);
      | port_label('input',si(1).port,si(1).txt);
      | port_label('input',si(2).port,si(2).txt);
      | 
      | port_label('output',so(1).port,so(1).txt);
      | port_label('output',so(2).port,so(2).txt);
  Template Matching : S-Function  FunctionName=sviptemplatematching  Parameters=metric,output,method,nMetric,nSize,roi,roiValid,dtInfo.prodOutputMode,dtInfo.prodOutputWordLength,dtInfo.prodOutputFracLength,dtInfo.accumMode,dtInfo.accumWordLength,dtInfo.accumFracLength,dtInfo.outputMode,dtInfo.outputWordLength,dtInfo.outputFracLength,dtInfo.roundingMode,dtInfo.overflowMode  SFunctionDeploymentMode=off  EnableBusSupport=off  mask(Template Matching){metric=Sum of absolute differences, output=Best match location, method=Exhaustive, nMetric=off, nSize=3, roi=off, roiValid=off, roundingMode=Floor, overflowMode=off, prodOutputMode=Binary point scaling, prodOutputWordLength=32, prodOutputFracLength=0, accumMode=Binary point scaling, accumWordLength=32, accumFracLength=0, outputMode=Same as first input, outputWordLength=32, outputFracLength=0, LockScale=off}
      mask prompts: metric "vision:masks:MatchMetric1"; output "vision:masks:Output1"; method "vision:masks:SearchMethod"; nMetric "vision:masks:OutputNxNMatrixOfMetricValues"; nSize "N:"; roi "vision:masks:EnableROIProcessing"; roiValid "vision:masks:OutputFlagIndicatingIfROIIsValid"; roundingMode "dspshared:FixptDialog:roundingMode"; overflowMode "Simulink:masks:SaturateOnIntegerOverflow_MP"; LockScale "Simulink:masks:LockDataTypeAgainstFxpTools_MP"
      mask help: vision:masks:TemplateMatchingDescription
      mask init:
      | [ports blkname]    = vipblktemplatematching('icon');
      | dtInfo   = vipblktemplatematching('init');
      mask Help: eval('visionblockhelp');
      mask TypeOptions metric: vision:masks:SumOfAbsoluteDifferences | vision:masks:SumOfSquaredDifferences | vision:masks:MaximumAbsoluteDifference
      mask Callback metric: vipblktemplatematching('dynamic')
      mask TypeOptions output: vision:masks:MetricMatrix | vision:masks:BestMatchLocation
      mask Callback output: vipblktemplatematching('dynamic')
      mask TypeOptions method: vision:masks:Exhaustive | vision:masks:Threestep
      mask Callback method: vipblktemplatematching('dynamic')
      mask Callback nMetric: vipblktemplatematching('dynamic')
      mask Callback nSize: vipblktemplatematching('dynamic')
      mask Callback roi: vipblktemplatematching('dynamic')
      mask Callback roiValid: vipblktemplatematching('dynamic')
      mask TypeOptions roundingMode: Simulink:dialog:Ceiling_CB | Simulink:dialog:Convergent_CB | Simulink:dialog:Floor_CB | Simulink:dialog:Nearest_CB | Simulink:dialog:Round_CB | Simulink:dialog:Simplest_CB | Simulink:dialog:Zero_CB
      mask TypeOptions prodOutputMode: Simulink:dialog:UDTSameAsFirstInputRule | vision:masks:BinaryPointScaling
      mask Callback prodOutputMode: vipblktemplatematching('dynamic')
      mask TypeOptions accumMode: Simulink:dialog:UDTSameAsFirstInputRule | vision:masks:BinaryPointScaling
      mask Callback accumMode: vipblktemplatematching('dynamic')
      mask TypeOptions outputMode: Simulink:dialog:UDTSameAsFirstInputRule | vision:masks:BinaryPointScaling
      mask Callback outputMode: vipblktemplatematching('dynamic')
      mask DialogControl MainTab Prompt: vision:masks:Main
      mask DialogControl metric Prompt: Match Metric:
      mask DialogControl OutputOptions Prompt: vision:masks:OutputOptions
      mask DialogControl output Prompt: Output:
      mask DialogControl method Prompt: Search method:
      mask DialogControl nMetric Prompt: Output NxN matrix of metric values around best match
      mask DialogControl ROIProcessing Prompt: vision:masks:ROIProcessing
      mask DialogControl roi Prompt: Enable ROI processing
      mask DialogControl roiValid Prompt: Output flag indicating if ROI is valid
      mask DialogControl DataTypesTab Prompt: Simulink:dialog:DataTypesTab
      mask DialogControl FloatingPointTrumpRule Prompt: Simulink:dialog:FloatingPointTrumpRule
      mask DialogControl FixPtOpParamsGroupBox Prompt: dspshared:FixptDialog:fixptOpParams
      mask DialogControl roundingMode Prompt: Rounding mode:
      mask DialogControl overflowMode Prompt: Saturate on integer overflow
      mask DialogControl FixptDatatypesGroupBox Prompt: dspshared:FixptDialog:fixptDataTypes
      mask DialogControl DataTypeColumnLabel Prompt: Simulink:dialog:BreakPointTableHeaderDT
      mask DialogControl SignedColumnLabel Prompt: dspshared:FixptDialog:signed
      mask DialogControl WordLengthColumnLabel Prompt: dspshared:FixptDialog:wordLength
      mask DialogControl FractionLengthColumnLabel Prompt: dspshared:FixptDialog:fractionLength
      mask DialogControl prodOutputLabel Prompt: Simulink:dialog:ProdPrompt
      mask DialogControl prodOutputSignedText Prompt: dspshared:FixptDialog:yes
      mask DialogControl accumLabel Prompt: Simulink:dialog:AccumPrompt
      mask DialogControl accumSignedText Prompt: Simulink:dialog:UDTSameAsInputRule
      mask DialogControl outputLabel Prompt: Simulink:dialog:OutputPrompt
      mask DialogControl outputSignedText Prompt: dspshared:FixptDialog:sameAsInput
      mask DialogControl LockScale Prompt: Lock data type settings against changes by the fixed-point tools
      mask Display:
      | disp(blkname)
      | port_label('input',ports.iport1, ports.itxt1);
      | port_label('input',ports.iport2, ports.itxt2);
      | port_label('input',ports.iport3, ports.itxt3);
      | port_label('output',ports.oport1, ports.otxt1);
      | port_label('output',ports.oport2, ports.otxt2);
      | port_label('output',ports.oport3, ports.otxt3);
      | port_label('output',ports.oport4, ports.otxt4);
  Trace Boundary : S-Function  FunctionName=sviptraceboundary  Parameters=conn,searchDir4,searchDir8,traceDir,maxNumPix,outputNum,fillChoices,fillVal  SFunctionDeploymentMode=off  EnableBusSupport=off  mask(Trace Boundary){conn=8, searchDir4=North, searchDir8=North, traceDir=Clockwise, maxNumPix=500, outputNum=off, fillChoices=None, fillVal=[0 0]}
      mask prompts: conn "vision:masks:Connectivity"; searchDir4 "vision:masks:InitialSearchDirection"; searchDir8 "vision:masks:InitialSearchDirection"; traceDir "vision:masks:TraceDirection"; maxNumPix "vision:masks:MaximumNumberOfBoundaryPixels"; outputNum "vision:masks:OutputNumberOfBoundaryPixels"; fillChoices "vision:masks:ActionToTakeForEmptyOutputPoints"; fillVal "vision:masks:FillValues"
      mask help: vision:masks:TraceBoundaryDescription
      mask init:
      | so = vipblkboundarytracing('icon2');
      mask Help: eval('visionblockhelp');
      mask TypeOptions conn: 4 | 8
      mask Callback conn: vipblkboundarytracing('dynamic2');
      mask TypeOptions searchDir4: vision:masks:North | vision:masks:East | vision:masks:South | vision:masks:West
      mask TypeOptions searchDir8: vision:masks:North | vision:masks:Northeast | vision:masks:East | vision:masks:Southeast | vision:masks:South | vision:masks:Southwest | vision:masks:West | vision:masks:Northwest
      mask TypeOptions traceDir: vision:masks:Clockwise | vision:masks:Counterclockwise
      mask TypeOptions fillChoices: vision:masks:None | vision:masks:FillWithLastPointFound | vision:masks:FillWithUserdefinedValues
      mask Display:
      | disp(['Trace\nBoundary']);
      | port_label('input',1,'BW');
      | port_label('input',2,'Start Pt');
      | port_label('output',so(1).port, so(1).txt);
      | port_label('output',so(2).port, so(2).txt);
